simulink library "videoStream_ul"  (R2018b)
settings: Solver=VariableStepAuto  StartTime=0.0  StopTime=10.0  RelTol=1e-3
libraries: visiongeotforms x1, xpcvideoutillib x1
settings Model: Creator=mcobb  LastModifiedBy=MAE-NCSUCORE
settings DebuggingCC: LibraryContextMissingDiagnostic=none
settings SFSimCC: SimUseLocalCustomCode=off
settings RTWCC: RTWUseLocalCustomCode=off

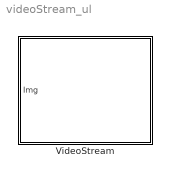
== system videoStream_ul ==
  VideoStream : Subsystem  TreatAsAtomicUnit=on  mask{enbl=on, decimationFactor=2, resizeFactor=1000}
      mask prompts: enbl "Enable"; decimationFactor "Video Sample Decimation"; resizeFactor "Display Image Width, num pixels"
      mask help:
      | Block to show video feed on target monitor.
      |
      | Enable : turns video feed on/off
      | Video Sample Decimation:  Should be a strictly positive integer, N.  Only update video feed every N time steps.  (eg Video Sample Decimation = 2 updates video on monitor every other time step).
      | Display Image Width: how wide, in pixels, is the image on the target screen.  Changing this does not reduce the resolution of the incoming image used in processing.
      | Note:  I'm not sure if decimation and display with can be tuned while the model is running.  You may have to stop and recompile for changes to take effect.  However, enable/disable works.  When disabled, display shows last captured image.
      | - MC 1/23/2019
      mask Display:
      | port_label('input',1,'Img')
      | 
      | enbl = get_param(gcb,'enbl');
      | 
      | if strcmpi(enbl,'on')
      |     color = [0 0.7 0];
      |     str = 'Enabled';
      | else
      |     color = [0.7 0 0];
      |     str = 'Disabled';
      | end
      | patch([0 1 1 0], [0.9 0.9 1 1],color)
      | 
      | str = [str '\nDecimation  = ' get_param(gcb,'decimationFactor') ];
      | str = [str '\nImage Width = ' get_param(gcb,'resizeFactor') ];
      | 
      | disp(str)

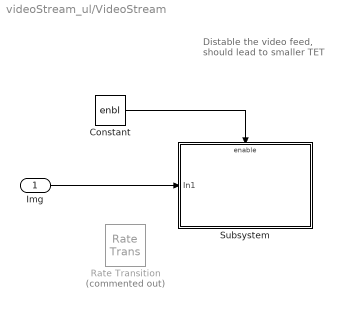
== system videoStream_ul/VideoStream ==
  note: Distable the video feed,
      | should lead to smaller TET
  Img : Inport
  Constant : Constant  Value=enbl
  Rate Transition : RateTransition  Commented=on  Deterministic=off  OutPortSampleTimeOpt=Multiple of input port sample time  OutPortSampleTimeMultiple=decimationFactor  OutPortSampleTime=0.05
  Subsystem : Subsystem
  wires:
  Img/1 -> Subsystem/1(In1)
  Constant/1 -> Subsystem/Enable

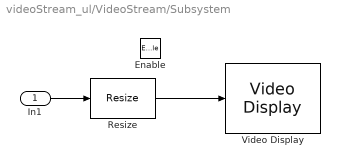
== system videoStream_ul/VideoStream/Subsystem ==
  In1 : Inport
  Enable : EnablePort
  Resize : visiongeotforms/Resize  specify=Number of output columns and preserve aspect ratio  rfactor=round(resizeFactor*[1 1])  outCols=round(resizeFactor);  outRows=25  outRowsCols=[25 35]  interp_method=Bilinear  antialias=on  useROI=off  roiFlag=off  prodOutputMode=Binary point scaling  prodOutputWordLength=32  prodOutputFracLength=10  roundingMode=Nearest  overflowMode=on
      settings: SourceProductName=Computer Vision System Toolbox  SourceProductBaseCode=VP
  Video Display : xpcvideoutillib/Video Display  imagesignal=Single multidimensional signal  colorspace=RGB  vindex=1  showpreview=on
      settings: SourceProductName=Simulink Real-Time  SourceProductBaseCode=XP
  wires:
  In1/1 -> Resize/1
  Resize/1 -> Video Display/1
